simulink model "differentialDriveRobot"  (R2024b)
settings: Solver=FixedStepAuto  StartTime=0.0  StopTime=10.0  FixedStep=0.001  RelTol=1e-3
values from neighbouring files (symbols this model uses):
  L = 0.5    [SimRun.m]
  R = 0.1    [SimRun.m]
settings Model: Creator=elija  LastModifiedBy=elija

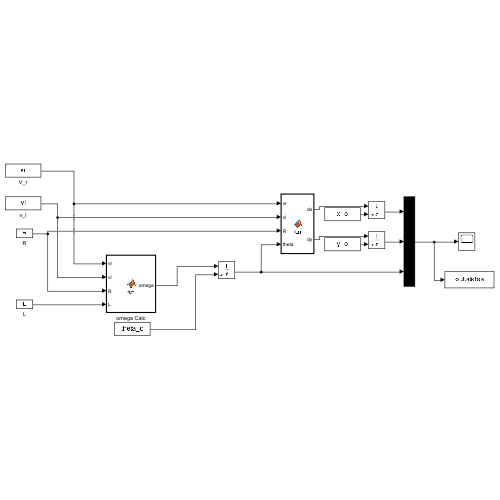
[thumbnail: Simulink's stored preview of the top-level diagram]
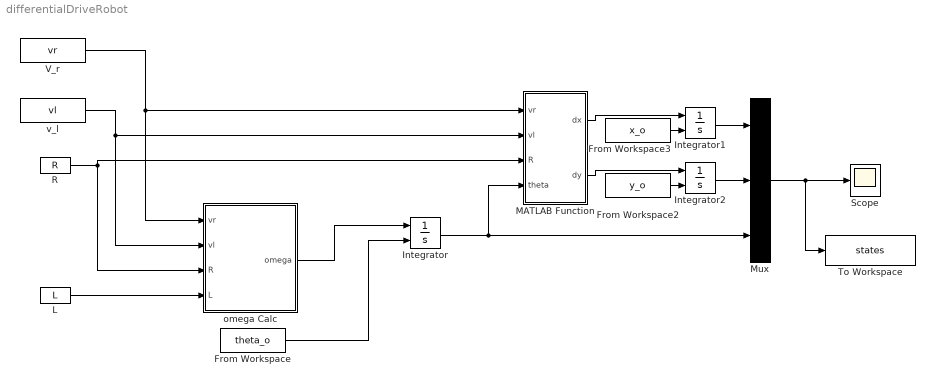
== system differentialDriveRobot ==
  From Workspace : FromWorkspace  VariableName=theta_o
  From Workspace2 : FromWorkspace  VariableName=y_o
  From Workspace3 : FromWorkspace  VariableName=x_o
  Integrator : Integrator  InitialConditionSource=external
  Integrator1 : Integrator  InitialConditionSource=external
  Integrator2 : Integrator  InitialConditionSource=external
  L : Constant  Value=L
  MATLAB Function : MATLAB Function  TreatAsAtomicUnit=on
  Mux : Mux  Inputs=3
  R : Constant  Value=R
  Scope : Scope
  To Workspace : ToWorkspace  VariableName=states  SaveFormat=Timeseries  SampleTime=-1
  V_r : FromWorkspace  VariableName=vr
  omega Calc : MATLAB Function  TreatAsAtomicUnit=on
  v_l : FromWorkspace  VariableName=vl
  wires:
  MATLAB Function/1(dx) -> Integrator1/1
  From Workspace/1 -> Integrator/2
  Integrator2/1 -> Mux/2
  From Workspace2/1 -> Integrator2/2
  Integrator/1 -> MATLAB Function/4(theta), Mux/3
  From Workspace3/1 -> Integrator1/2
  MATLAB Function/2(dy) -> Integrator2/1
  Mux/1 -> To Workspace/1, Scope/1
  Integrator1/1 -> Mux/1
  omega Calc/1(omega) -> Integrator/1
  L/1 -> omega Calc/4(L)
  R/1 -> MATLAB Function/3(R), omega Calc/3(R)
  V_r/1 -> omega Calc/1(vr), MATLAB Function/1(vr)
  v_l/1 -> omega Calc/2(vl), MATLAB Function/2(vl)

== matlab function differentialDriveRobot/omega Calc ==
  data: vr input; omega output; vl input; R input; L input
function omega = fcn(vr,vl,R,L)
omega = (R./L).*(vr-vl);
end

== matlab function differentialDriveRobot/MATLAB Function ==
  data: dx output; dy output; vr input; vl input; R input; theta input
function [dx,dy] = fcn(vr,vl,R,theta)

dy = (R./2).*(vr+vl).*sin(theta);
dx = (R./2).*(vr+vl).*cos(theta);

end
